simulink model "ZRM_2_STATES"  (R2016a)
settings: Solver=VariableStepAuto  StartTime=0.0  StopTime=100  FixedStep=0.01  RelTol=1e-2
values from neighbouring files (symbols this model uses):
  u_AP = [0 0 0]    [Computation_Two_States.m]
  x_0 = [0 0 0 0]    [Computation_Two_States.m]
  x_AP = [0 0 0 0]    [Computation_Two_States.m]
undefined symbols (not defined in the file or in its folder): alpha, beta, K
libraries: simulink x1
settings Model: Creator=Florian  LastModifiedBy=Florian

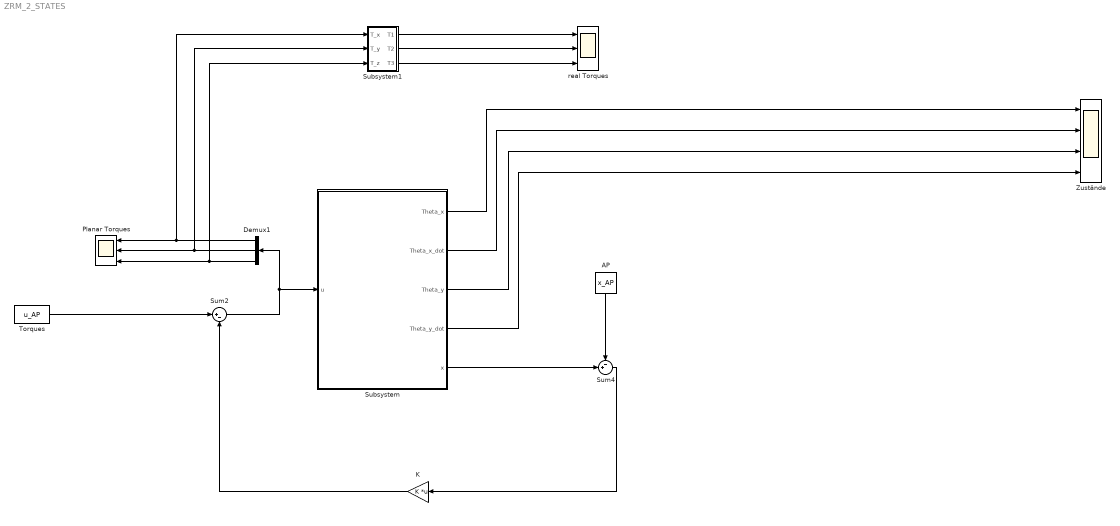
== system ZRM_2_STATES ==
  "AP " : Constant  Value=x_AP
  Demux1 : Demux  Outputs=3
  K : Gain  Gain=K  Multiplication=Matrix(K*u)
  Planar Torques : Scope  NumInputPorts=3
  Subsystem : Subsystem
  Subsystem1 : Subsystem
  Sum2 : Sum  Inputs=|+-
  Sum4 : Sum  Inputs=-+|
  "Torques " : Constant  Value=u_AP
  "Zustände " : Scope  NumInputPorts=4
  "real Torques " : Scope  NumInputPorts=3
  wires:
  "Torques "/1 -> Sum2/1
  Subsystem/5(x) -> Sum4/2
  "AP "/1 -> Sum4/1
  K/1 -> Sum2/2
  Subsystem/1(Theta_x) -> "Zustände "/1
  Subsystem/2(Theta_x_dot) -> "Zustände "/2
  Subsystem/3(Theta_y) -> "Zustände "/3
  Subsystem/4(Theta_y_dot) -> "Zustände "/4
  Demux1/1 -> Planar Torques/1, Subsystem1/1(T_x)
  Demux1/2 -> Planar Torques/2, Subsystem1/2(T_y)
  Demux1/3 -> Subsystem1/3(T_z), Planar Torques/3
  Subsystem1/1(T1) -> "real Torques "/1
  Subsystem1/2(T2) -> "real Torques "/2
  Subsystem1/3(T3) -> "real Torques "/3
  Sum2/1 -> Subsystem/1("u "), Demux1/1
  Sum4/1 -> K/1

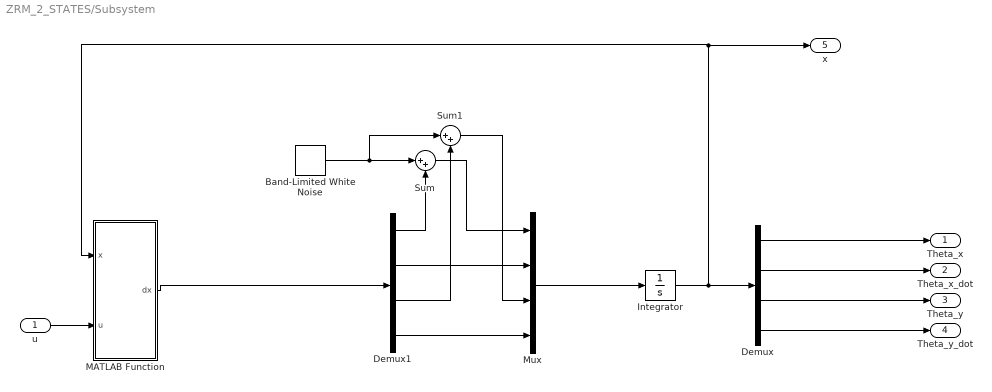
== system ZRM_2_STATES/Subsystem ==
  "u " : Inport
  Band-Limited White Noise : simulink/Sources/Band-Limited White Noise  Cov=[0.1^2]  Ts=1/100  seed=[23341]
  Demux : Demux
  Demux1 : Demux
  Integrator : Integrator  InitialCondition=x_0
  MATLAB Function : MATLAB Function  TreatAsAtomicUnit=on
  Mux : Mux
  Sum : Sum  Inputs=|++
  Sum1 : Sum  Inputs=|++
  Theta_x : Outport
  Theta_x_dot : Outport  Port=2
  Theta_y : Outport  Port=3
  Theta_y_dot : Outport  Port=4
  x : Outport  Port=5
  wires:
  MATLAB Function/1(dx) -> Demux1/1
  Band-Limited White Noise/1 -> Sum1/1, Sum/1
  Integrator/1 -> Demux/1, MATLAB Function/1(x), x/1
  Sum/1 -> Mux/1
  Demux1/3 -> Sum1/2
  Mux/1 -> Integrator/1
  Demux1/1 -> Sum/2
  Sum1/1 -> Mux/3
  Demux1/4 -> Mux/4
  Demux1/2 -> Mux/2
  Demux/3 -> Theta_y/1
  Demux/1 -> Theta_x/1
  Demux/2 -> Theta_x_dot/1
  Demux/4 -> Theta_y_dot/1
  "u "/1 -> MATLAB Function/2(u)

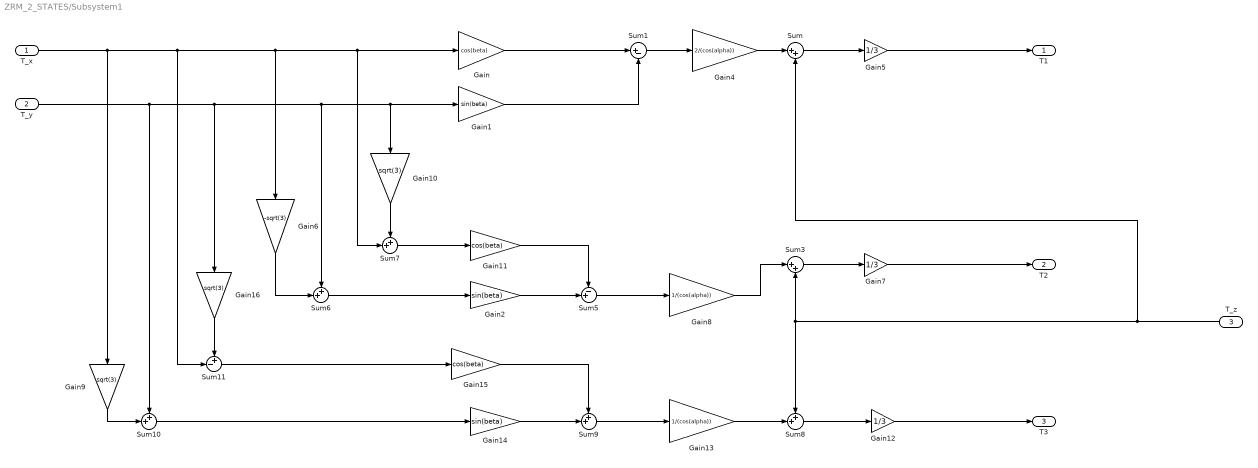
== system ZRM_2_STATES/Subsystem1 ==
  T_x : Inport
  T_y : Inport  Port=2
  T_z : Inport  Port=3
  Gain : Gain  Gain=cos(beta)
  Gain1 : Gain  Gain=sin(beta)
  Gain10 : Gain  Gain=sqrt(3)
  Gain11 : Gain  Gain=cos(beta)
  Gain12 : Gain  Gain=1/3
  Gain13 : Gain  Gain=1/(cos(alpha))
  Gain14 : Gain  Gain=sin(beta)
  Gain15 : Gain  Gain=cos(beta)
  Gain16 : Gain  Gain=sqrt(3)
  Gain2 : Gain  Gain=sin(beta)
  Gain4 : Gain  Gain=2/(cos(alpha))
  Gain5 : Gain  Gain=1/3
  Gain6 : Gain  Gain=-sqrt(3)
  Gain7 : Gain  Gain=1/3
  Gain8 : Gain  Gain=1/(cos(alpha))
  Gain9 : Gain  Gain=sqrt(3)
  Sum : Sum  Inputs=|++
  Sum1 : Sum  Inputs=|+-
  Sum{6..10} (5 alike) : Sum  Inputs=++|
  Sum11 : Sum  Inputs=+-|
  Sum3 : Sum  Inputs=|++
  Sum5 : Sum  Inputs=-+|
  T1 : Outport
  T2 : Outport  Port=2
  T3 : Outport  Port=3
  wires:
  Sum1/1 -> Gain4/1
  Sum7/1 -> Gain11/1
  Gain13/1 -> Sum8/2
  Gain10/1 -> Sum7/1
  Gain4/1 -> Sum/1
  Sum11/1 -> Gain15/1
  Gain5/1 -> T1/1
  T_y/1 -> Gain16/1, Gain1/1, Gain10/1, Sum6/1, Sum10/1
  T_x/1 -> Sum11/2, Gain/1, Sum7/2, Gain6/1, Gain9/1
  Gain11/1 -> Sum5/1
  Sum9/1 -> Gain13/1
  Gain12/1 -> T3/1
  Sum8/1 -> Gain12/1
  Gain8/1 -> Sum3/1
  Gain15/1 -> Sum9/1
  Sum10/1 -> Gain14/1
  Sum6/1 -> Gain2/1
  Gain9/1 -> Sum10/2
  Gain7/1 -> T2/1
  Gain14/1 -> Sum9/2
  Gain6/1 -> Sum6/2
  Gain2/1 -> Sum5/2
  T_z/1 -> Sum3/2, Sum8/1, Sum/2
  Gain16/1 -> Sum11/1
  Sum/1 -> Gain5/1
  Gain1/1 -> Sum1/2
  Sum5/1 -> Gain8/1
  Gain/1 -> Sum1/1
  Sum3/1 -> Gain7/1

== matlab function ZRM_2_STATES/Subsystem/MATLAB Function ==
  data: x input; dx output; u input
function dx = fcn(x,u)

T_x = u(1);
T_y = u(2);
T_z = u(3);

theta_x = x(1);
theta_x_dot = x(2);
theta_y = x(3);
theta_y_dot = x(4);
 
theta_x_dotdot = (6016648984670743898930240217415680*T_x + 29524150483558187301665611373107008*sin(theta_x) + 289041203960050657418688165988680*theta_x_dot^2*sin(theta_x) - 1472871455302348959855892773208064*T_x*cos(theta_x) - 19184770784195777962831677291729*theta_x_dot^2*cos(theta_x)*sin(theta_x))/(9*(64231378657789034981930703553040*cos(theta_x) - 2131641198243975329203519699081*cos(theta_x)^2 + 163980781556649271175210059272000)); 
theta_y_dotdot = (6016648984670743898930240217415680*T_y + 29524150483558187301665611373107008*sin(theta_y) + 289041203960050657418688165988680*theta_y_dot^2*sin(theta_y) - 1472871455302348959855892773208064*T_y*cos(theta_y) - 19184770784195777962831677291729*theta_y_dot^2*cos(theta_y)*sin(theta_y))/(9*(64231378657789034981930703553040*cos(theta_y) - 2131641198243975329203519699081*cos(theta_y)^2 + 163980781556649271175210059272000));  

dx = [theta_x_dot, theta_x_dotdot, theta_y_dot, theta_y_dotdot];
